simulink model "ans3_65070121_155_168"  (R2024b)
settings: Solver=VariableStepAuto  StartTime=0.0  StopTime=5  RelTol=1e-3
settings Model: Creator=picha  LastModifiedBy=picha

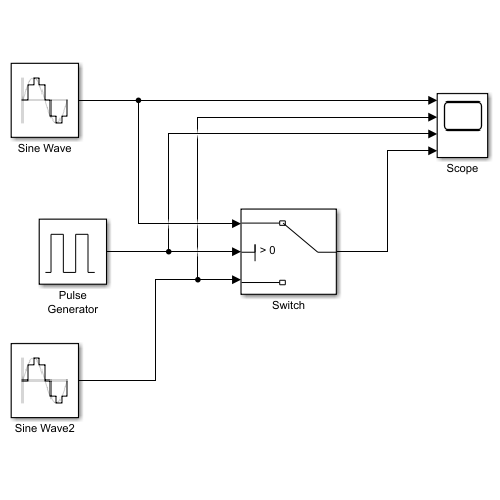
[thumbnail: Simulink's stored preview of the top-level diagram]
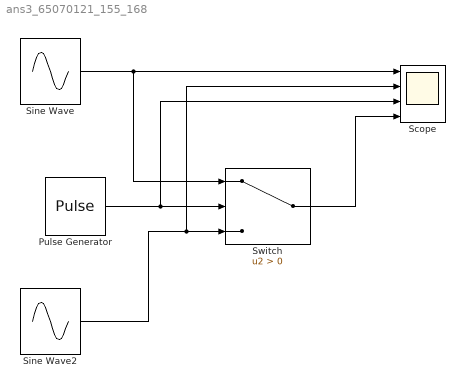
== system ans3_65070121_155_168 ==
  Pulse Generator : DiscretePulseGenerator  PulseType=Time based  PulseWidth=50
  Scope : Scope  NumInputPorts=4
  Sine Wave : Sin  Frequency=2*pi  SampleTime=0.001
  Sine Wave2 : Sin  Frequency=4*pi  SampleTime=0.001
  Switch : Switch  Criteria=u2 > Threshold  SaturateOnIntegerOverflow=off  InputSameDT=off
  wires:
  Sine Wave/1 -> Switch/1, Scope/1
  Pulse Generator/1 -> Scope/3, Switch/2
  Switch/1 -> Scope/4
  Sine Wave2/1 -> Scope/2, Switch/3
